simulink library "lib_dsphdldsp_v1"  (R2019b)
settings: Solver=VariableStepAuto  StartTime=0.0  StopTime=10.0  RelTol=1e-3
libraries: simulink x2
settings Model: Creator=mbabst  LastModifiedBy=mbabst
settings DebuggingCC: ArithmeticOperatorsInVariantConditions=warning
settings SFSimCC: SimUseLocalCustomCode=off  CustomCodeUndefinedFunction=UseInterfaceOnly
settings RTWCC: RTWUseLocalCustomCode=off
settings CodeAppCC: StateflowObjectComments=on

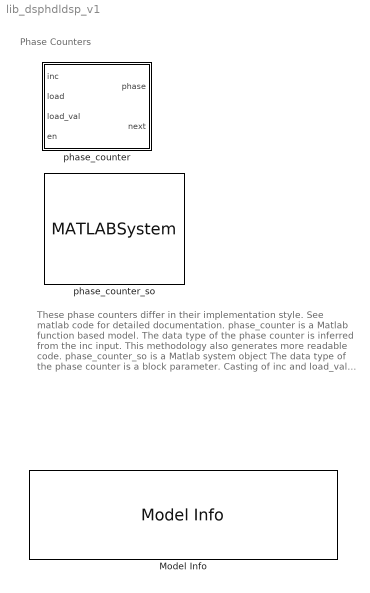
== system lib_dsphdldsp_v1 ==
  note: These phase counters differ in their implementation style.
      | See matlab code for detailed documentation.
      |
      | phase_counter is a Matlab function based model.
      | The data type of the phase counter is inferred from the inc input.
      | This methodology also generates more readable code.
      |
      | phase_counter_so is a Matlab system object
      | The data type of the phase counter is a block parameter.
      | Casting of inc and load_val is done internally.
      | This methodology generates less readable code.
  note: Phase Counters
  Model Info : simulink/Model-Wide Utilities/Model Info  Frame=on  DisplayStringWithTags=|  HorizontalTextAlignment=Left  LeftAlignmentValue=0.02
      | Copyright (c) 2005-2021 DSPlogic, Inc.
      | Distributed under the terms of the Simplified BSD License.
      | The full license is in the file LICENSE, distributed with this software.
      | 
      | Model: %<ModelName> (v%<ModelVersion>)
      | Author: Michael Babst <mike.babst@dsplogic.com>
      | Created: by %<Creator> on %<Created>
      | Modified: by %<ModifiedBy> on %<LastModificationDate>
  phase_counter : Subsystem
  phase_counter_so : MATLABSystem  System=phase_counter_so  WordLength=8  SimulateUsing=Code generation
      mask Type: phase_counter_so
      mask Display:
      | disp('phase_counter_so');
      | port_label('input',1,'en');
      | port_label('input',2,'inc');
      | port_label('input',3,'load');
      | port_label('input',4,'load_val');
      | port_label('output',1,'phase');
      | port_label('output',2,'next');

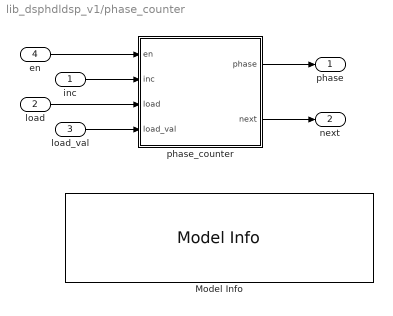
== system lib_dsphdldsp_v1/phase_counter ==
  inc : Inport
  load : Inport  Port=2
  load_val : Inport  Port=3
  en : Inport  Port=4
  Model Info : simulink/Model-Wide Utilities/Model Info  Frame=on  DisplayStringWithTags=|  HorizontalTextAlignment=Left  LeftAlignmentValue=0.02
      | Copyright (c) 2005-2021 DSPlogic, Inc.
      | Distributed under the terms of the Simplified BSD License.
      | The full license is in the file LICENSE, distributed with this software.
      | 
      | Model: %<ModelName> (v%<ModelVersion>)
      | Author: Michael Babst <mike.babst@dsplogic.com>
      | Created: by %<Creator> on %<Created>
      | Modified: by %<ModifiedBy> on %<LastModificationDate>
  phase_counter : MATLAB Function  TreatAsAtomicUnit=on
  phase : Outport
  next : Outport  Port=2
  wires:
  inc/1 -> phase_counter/2(inc)
  phase_counter/1(phase) -> phase/1
  load/1 -> phase_counter/3(load)
  load_val/1 -> phase_counter/4(load_val)
  phase_counter/2(next) -> next/1
  en/1 -> phase_counter/1(en)

== matlab function lib_dsphdldsp_v1/phase_counter/phase_counter ==
  data: en input; inc input; phase output; load input; load_val input; next output
%#codegen
function [ phase, next ] = phase_counter( en, inc, load, load_val )

[ phase, next ] = phase_counter( en, inc, load, load_val );
